simulink model "sim_closedloop"  (R2024b)
settings: Solver=VariableStepAuto  StartTime=0.0  StopTime=simulation_time  RelTol=1e-3
values from neighbouring files (symbols this model uses):
  age = 18    [main_sim_closedloop.m]
  gender = 0    [main_sim_closedloop.m]
  height = 170    [main_sim_closedloop.m]
  Kp = 0.0286    [main_sim_closedloop.m]
  N = 5    [main_sim_closedloop.m]
  ratio = 2    [main_sim_closedloop.m]
  sampling_time = 1    [main_sim_closedloop.m]
  sat_neg_p = 0    [main_sim_closedloop.m]
  sat_neg_r = 0    [main_sim_closedloop.m]
  sat_pos_p = 6.67    [main_sim_closedloop.m]
  sat_pos_r = 16.67    [main_sim_closedloop.m]
  Td = 29.83    [main_sim_closedloop.m]
  Ti = 206.98    [main_sim_closedloop.m]
  Ts = 5    [main_sim_closedloop.m]
  uref_p = 0    [main_sim_closedloop.m]
  uref_r = 0    [main_sim_closedloop.m]
  weight = 60    [main_sim_closedloop.m]
settings Model: Creator=michele.schiavo  LastModifiedBy=michele.schiavo

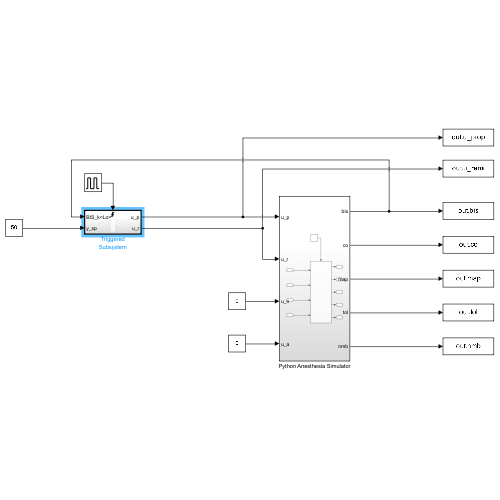
[thumbnail: Simulink's stored preview of the top-level diagram]
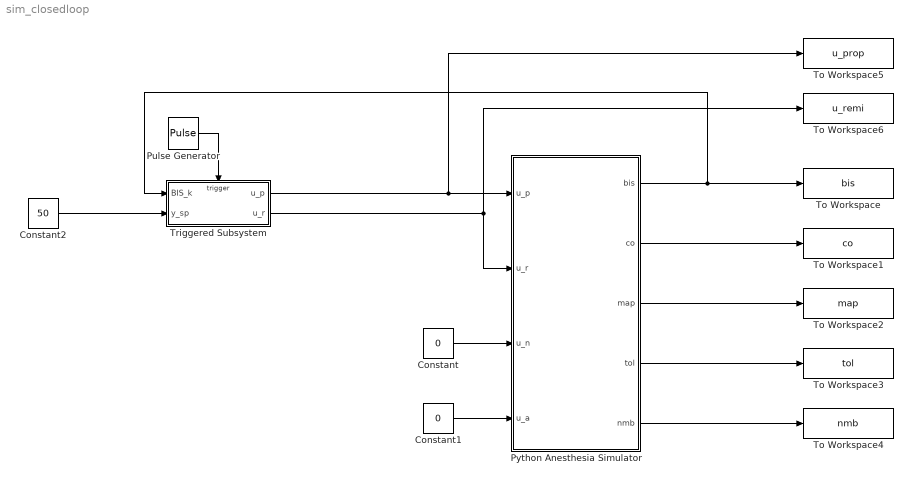
== system sim_closedloop ==
  Constant : Constant  Value=0
  Constant1 : Constant  Value=0
  Constant2 : Constant  Value=50
  Pulse Generator : DiscretePulseGenerator  PulseType=Time based  Period=Ts  PulseWidth=5
  Python Anesthesia Simulator : Subsystem
  To Workspace : ToWorkspace  VariableName=bis  SaveFormat=Timeseries  SampleTime=-1
  To Workspace1 : ToWorkspace  VariableName=co  SaveFormat=Timeseries  SampleTime=-1
  To Workspace2 : ToWorkspace  VariableName=map  SaveFormat=Timeseries  SampleTime=-1
  To Workspace3 : ToWorkspace  VariableName=tol  SaveFormat=Timeseries  SampleTime=-1
  To Workspace4 : ToWorkspace  VariableName=nmb  SaveFormat=Timeseries  SampleTime=-1
  To Workspace5 : ToWorkspace  VariableName=u_prop  SaveFormat=Timeseries  SampleTime=-1
  To Workspace6 : ToWorkspace  VariableName=u_remi  SaveFormat=Timeseries  SampleTime=-1
  Triggered Subsystem : Subsystem  TreatAsAtomicUnit=on
  wires:
  Triggered Subsystem/1(u_p) -> To Workspace5/1, Python Anesthesia Simulator/1(u_p)
  Python Anesthesia Simulator/1(bis) -> Triggered Subsystem/1(BIS_k), To Workspace/1
  Triggered Subsystem/2(u_r) -> Python Anesthesia Simulator/2(u_r), To Workspace6/1
  Constant/1 -> Python Anesthesia Simulator/3(u_n)
  Constant1/1 -> Python Anesthesia Simulator/4(u_a)
  Python Anesthesia Simulator/2(co) -> To Workspace1/1
  Python Anesthesia Simulator/3(map) -> To Workspace2/1
  Python Anesthesia Simulator/4(tol) -> To Workspace3/1
  Python Anesthesia Simulator/5(nmb) -> To Workspace4/1
  Pulse Generator/1 -> Triggered Subsystem/Trigger
  Constant2/1 -> Triggered Subsystem/2(y_sp)

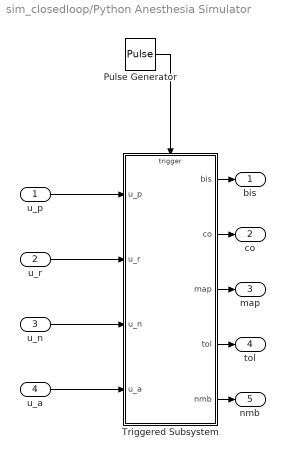
== system sim_closedloop/Python Anesthesia Simulator ==
  u_p : Inport
  u_r : Inport  Port=2
  u_n : Inport  Port=3
  u_a : Inport  Port=4
  Pulse Generator : DiscretePulseGenerator  PulseType=Time based  Period=sampling_time  PulseWidth=5
  Triggered Subsystem : Subsystem  TreatAsAtomicUnit=on
  bis : Outport
  co : Outport  Port=2
  map : Outport  Port=3
  tol : Outport  Port=4
  nmb : Outport  Port=5
  wires:
  Pulse Generator/1 -> Triggered Subsystem/Trigger
  Triggered Subsystem/3(map) -> map/1
  u_p/1 -> Triggered Subsystem/1(u_p)
  Triggered Subsystem/4(tol) -> tol/1
  Triggered Subsystem/2(co) -> co/1
  Triggered Subsystem/1(bis) -> bis/1
  Triggered Subsystem/5(nmb) -> nmb/1
  u_r/1 -> Triggered Subsystem/2(u_r)
  u_n/1 -> Triggered Subsystem/3(u_n)
  u_a/1 -> Triggered Subsystem/4(u_a)

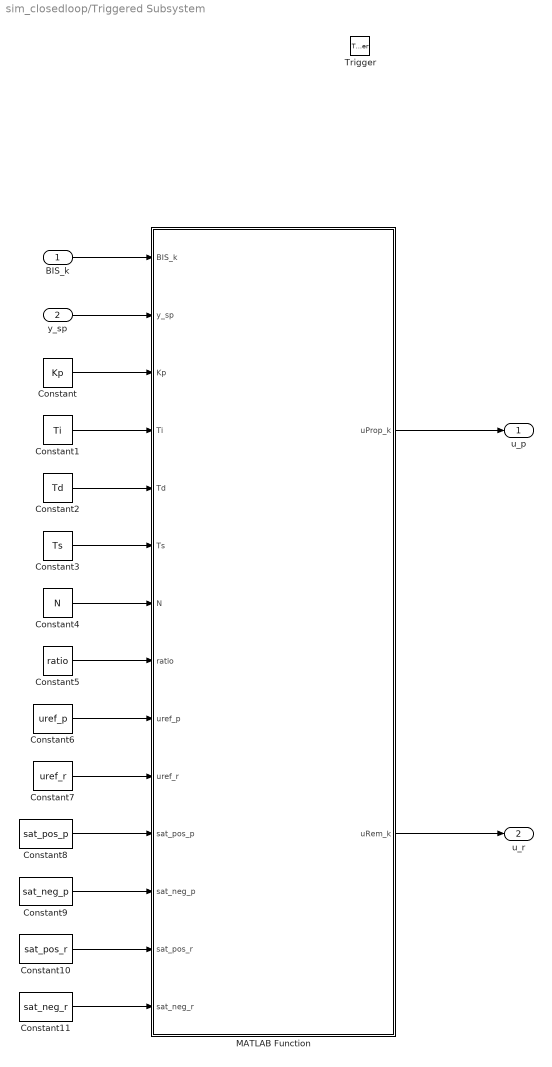
== system sim_closedloop/Triggered Subsystem ==
  BIS_k : Inport  LatchByDelayingOutsideSignal=on
  y_sp : Inport  Port=2
  Trigger : TriggerPort  VariantControl=(inherit)
  Constant : Constant  Value=Kp
  Constant1 : Constant  Value=Ti
  Constant10 : Constant  Value=sat_pos_r
  Constant11 : Constant  Value=sat_neg_r
  Constant2 : Constant  Value=Td
  Constant3 : Constant  Value=Ts
  Constant4 : Constant  Value=N
  Constant5 : Constant  Value=ratio
  Constant6 : Constant  Value=uref_p
  Constant7 : Constant  Value=uref_r
  Constant8 : Constant  Value=sat_pos_p
  Constant9 : Constant  Value=sat_neg_p
  MATLAB Function : MATLAB Function  TreatAsAtomicUnit=on
  u_p : Outport
  u_r : Outport  Port=2
  wires:
  BIS_k/1 -> MATLAB Function/1(BIS_k)
  y_sp/1 -> MATLAB Function/2(y_sp)
  MATLAB Function/1(uProp_k) -> u_p/1
  MATLAB Function/2(uRem_k) -> u_r/1
  Constant/1 -> MATLAB Function/3(Kp)
  Constant1/1 -> MATLAB Function/4(Ti)
  Constant2/1 -> MATLAB Function/5(Td)
  Constant3/1 -> MATLAB Function/6(Ts)
  Constant4/1 -> MATLAB Function/7(N)
  Constant5/1 -> MATLAB Function/8(ratio)
  Constant6/1 -> MATLAB Function/9(uref_p)
  Constant7/1 -> MATLAB Function/10(uref_r)
  Constant8/1 -> MATLAB Function/11(sat_pos_p)
  Constant9/1 -> MATLAB Function/12(sat_neg_p)
  Constant10/1 -> MATLAB Function/13(sat_pos_r)
  Constant11/1 -> MATLAB Function/14(sat_neg_r)

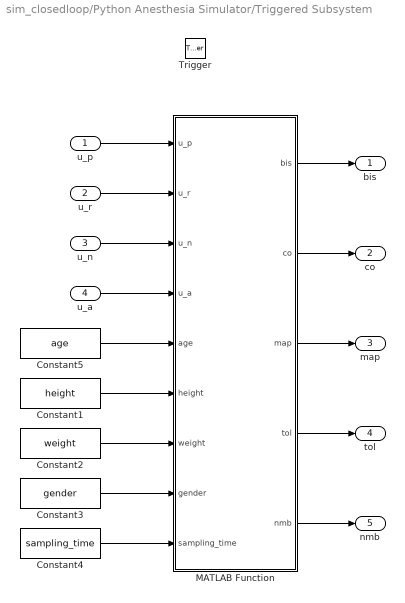
== system sim_closedloop/Python Anesthesia Simulator/Triggered Subsystem ==
  u_p : Inport
  u_r : Inport  Port=2
  u_n : Inport  Port=3
  u_a : Inport  Port=4
  Trigger : TriggerPort  VariantControl=(inherit)
  Constant1 : Constant  Value=height
  Constant2 : Constant  Value=weight
  Constant3 : Constant  Value=gender
  Constant4 : Constant  Value=sampling_time
  Constant5 : Constant  Value=age
  MATLAB Function : MATLAB Function  TreatAsAtomicUnit=on
  bis : Outport
  co : Outport  Port=2
  map : Outport  Port=3
  tol : Outport  Port=4
  nmb : Outport  Port=5
  wires:
  u_p/1 -> MATLAB Function/1(u_p)
  MATLAB Function/1(bis) -> bis/1
  u_r/1 -> MATLAB Function/2(u_r)
  MATLAB Function/2(co) -> co/1
  MATLAB Function/3(map) -> map/1
  MATLAB Function/4(tol) -> tol/1
  MATLAB Function/5(nmb) -> nmb/1
  u_n/1 -> MATLAB Function/3(u_n)
  u_a/1 -> MATLAB Function/4(u_a)
  Constant5/1 -> MATLAB Function/5(age)
  Constant1/1 -> MATLAB Function/6(height)
  Constant2/1 -> MATLAB Function/7(weight)
  Constant3/1 -> MATLAB Function/8(gender)
  Constant4/1 -> MATLAB Function/9(sampling_time)

== matlab function sim_closedloop/Triggered Subsystem/MATLAB Function ==
  data: BIS_k input; uProp_k output; y_sp input; Kp input; Ti input; Td input; Ts input; N input; ratio input; uref_p input; uref_r input; sat_pos_p input; sat_neg_p input; sat_pos_r input; sat_neg_r input; uRem_k output
function [uProp_k, uRem_k] = pid_ratio(BIS_k, y_sp, Kp, Ti, Td, Ts, N, ratio, uref_p, uref_r, sat_pos_p, sat_neg_p, sat_pos_r, sat_neg_r)
% PID_RATIO A PID controller for propofol and remifentanil ratio
% coadministration with saturation and anti-windup
%
% Inputs:
%   BIS_k   - Current BIS value
%   y_sp    - Setpoint for BIS
%   parameters:
%       Kp, Ti, Td, Ts, N              : PID tuning parameters
%       ratio                          : Remifentanil/propofol ratio
%       uref_p, uref_r                 : Baseline infusion rates
%       sat_pos_p, sat_neg_p           : Saturation limits for propofol
%       sat_pos_r, sat_neg_r           : Saturation limits for remifentanil
%
% Outputs:
%   uProp_k - Control input for propofol
%   uRem_k  - Control input for remifentanil

    persistent y_k1 ei_k1 d_k1 i_k1 init

    if isempty(init)
        y_k1 = BIS_k;
        ei_k1 = 0;
        d_k1 = 0;
        i_k1 = 0;
        init = true;
    end


    % PID error and terms
    e_k = BIS_k - y_sp;
    i_k = (Kp*Ts*ei_k1 + Ti*i_k1) / Ti;
    d_k = (2*Td*N*Kp*BIS_k - 2*Td*N*Kp*y_k1 - (Ts*N - 2*Td)*d_k1) /...
        (Ts*N + 2*Td);
    p_k = Kp*e_k;
    u_k = p_k + i_k + d_k;

    % Apply baseline offsets
    u_k_p = u_k + uref_p;
    u_k_r = (u_k*ratio) + uref_r;

    % Saturation logic
    if u_k_p > sat_pos_p
        u_sat_p = sat_pos_p;
        sat_k_p = 1;
    elseif u_k_p < sat_neg_p
        u_sat_p = sat_neg_p;
        sat_k_p = 1;
    else
        u_sat_p = u_k_p;
        sat_k_p = 0;
    end

    if u_k_r > sat_pos_r
        u_sat_r = sat_pos_r;
        sat_k_r = 1;
    elseif u_k_r < sat_neg_r
        u_sat_r = sat_neg_r;
        sat_k_r = 1;
    else
        u_sat_r = u_k_r;
        sat_k_r = 0;
    end

    % Anti-windup: clip integral if saturation occurred
    if sat_k_p || sat_k_r
        ei_k1 = 0;
    else
        ei_k1 = e_k;
    end

    % Update memory
    y_k1 = BIS_k;
    d_k1 = d_k;
    i_k1 = i_k;

    % Output
    uProp_k = u_sat_p;
    uRem_k  = u_sat_r;
end

== matlab function sim_closedloop/Python Anesthesia Simulator/Triggered Subsystem/MATLAB Function ==
  data: u_p input; bis output; u_r input; u_n input; u_a input; co output; map output; tol output; nmb output; age input; height input; weight input; gender input; sampling_time input
function [bis, co, map, tol, nmb] = PythonStep(u_p,u_r,u_n,u_a,age,height,weight,gender,sampling_time)
    coder.extrinsic('callPython')
    % Default value for codegen
    bis = 0; 
    co = 0;
    map = 0;
    tol = 0;
    nmb = 0;
    [bis, co, map, tol, nmb] = callPython(u_p,u_r,u_n,u_a,age,height,weight,gender,sampling_time);
end
